simulink model "singlecomponent_SWC_InpMgmt_AFE"  (R2022b)
settings: configuration reference "DC_DC_Charger_Configuration" (kept outside this file)
libraries: common_lib x2
settings Model: DataDictionary=SWC_InpMgmt_AFE.sldd  SimulationMode=accelerator  ExtModeTrigDuration=8  Creator=E0654638  LastModifiedBy=E0660158
settings ConfigSetRef: SourceName=DC_DC_Charger_Configuration

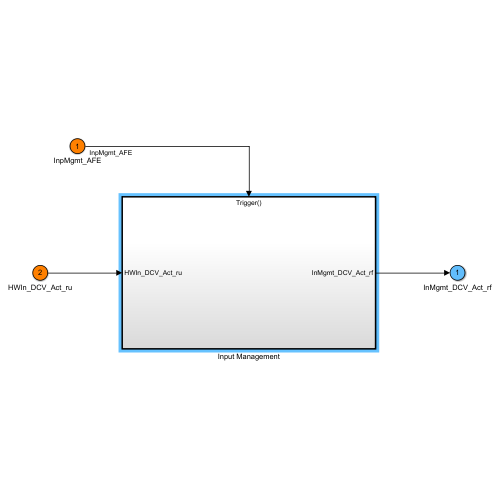
[thumbnail: Simulink's stored preview of the top-level diagram]
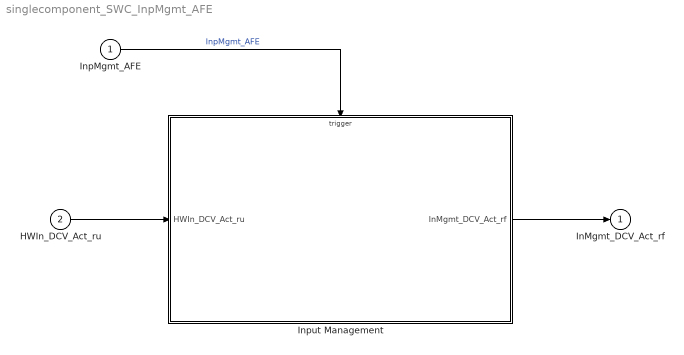
== system singlecomponent_SWC_InpMgmt_AFE ==
  InpMgmt_AFE : Inport  Description=Inverter HVDC voltage  OutMin=0  OutMax=1000  PortDimensions=1  SampleTime=2.5e-5  OutputFunctionCall=on
  HWIn_DCV_Act_ru : Inport  Port=2  OutDataTypeStr=uint16
  Input Management : Subsystem
  InMgmt_DCV_Act_rf : Outport  OutDataTypeStr=single  VectorParamsAs1DForOutWhenUnconnected=off
  wires:
  InpMgmt_AFE/1 -> Input Management/Trigger  "InpMgmt_AFE"
  HWIn_DCV_Act_ru/1 -> Input Management/1(HWIn_DCV_Act_ru)
  Input Management/1(InMgmt_DCV_Act_rf) -> InMgmt_DCV_Act_rf/1

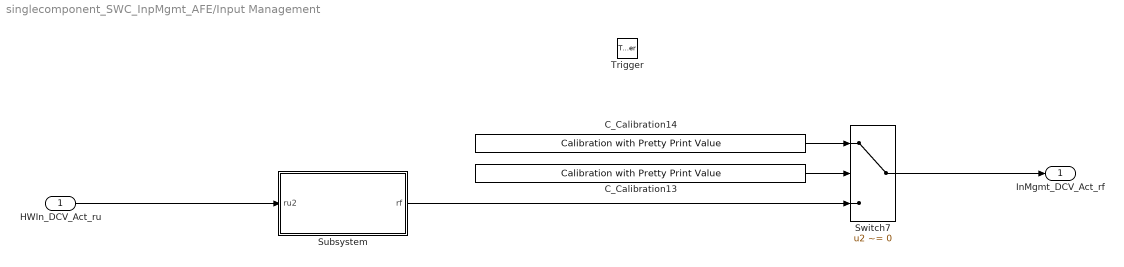
== system singlecomponent_SWC_InpMgmt_AFE/Input Management ==
  HWIn_DCV_Act_ru : Inport
  Trigger : TriggerPort  TriggerType=function-call  VariantControl=(inherit)  SampleTimeType=periodic  SampleTime=-1  PortDimensions=1
  C_Calibration13 : common_lib/IO/Calibration with Pretty Print Value  CalValue=InpMgmt_DCV_Act_ru_TO  scaling=None
      settings: SourceProductName=Common Library Blocks
  C_Calibration14 : common_lib/IO/Calibration with Pretty Print Value  CalValue=InpMgmt_DCV_Act_ru_TC  scaling=None
      settings: SourceProductName=Common Library Blocks
  Subsystem : Subsystem
  Switch7 : Switch  Criteria=u2 ~= 0  SaturateOnIntegerOverflow=off  InputSameDT=off
  InMgmt_DCV_Act_rf : Outport
  wires:
  HWIn_DCV_Act_ru/1 -> Subsystem/1(ru2)
  Switch7/1 -> InMgmt_DCV_Act_rf/1
  Subsystem/1(rf) -> Switch7/3
  C_Calibration13/1 -> Switch7/2
  C_Calibration14/1 -> Switch7/1

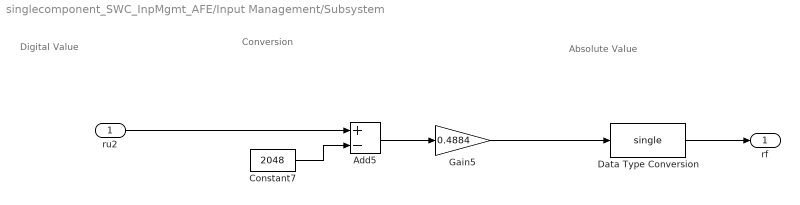
== system singlecomponent_SWC_InpMgmt_AFE/Input Management/Subsystem ==
  note: Absolute Value
  note: Digital Value
  note: Conversion
  ru2 : Inport
  Add5 : Sum  Inputs=+-  OutDataTypeStr=uint16
  Constant7 : Constant  Value=2048  OutDataTypeStr=uint16
  Data Type Conversion : DataTypeConversion  OutDataTypeStr=single  SaturateOnIntegerOverflow=off  RndMeth=Floor
  Gain5 : Gain  Gain=0.4884  OutDataTypeStr=uint16
  rf : Outport
  wires:
  Gain5/1 -> Data Type Conversion/1
  ru2/1 -> Add5/1
  Constant7/1 -> Add5/2
  Add5/1 -> Gain5/1
  Data Type Conversion/1 -> rf/1
